simulink model "LCK_0112"  (R2018b)
settings: Solver=FixedStepDiscrete  StartTime=0.0  StopTime=inf  FixedStep=0.01  RelTol=1e-3
PostLoadFcn:
  | if any(exist('dsrtsu_mdlpostloadfcn', 'file') ~= 0), dsrtsu_mdlpostloadfcn('Execute', bdroot); end
values from neighbouring files (symbols this model uses):
  C_DEG2RAD = 0.0175    [LCK_Macro.sldd]
  C_KPH2MPS = 0.2778    [LCK_Macro.sldd]
  C_NEARZERO = 0.0001    [LCK_Macro.sldd]
  C_ONE = 1.0    [LCK_Macro.sldd]
  C_RAD2DEG = 57.2958    [LCK_Macro.sldd]
  C_ZERO = 0.0    [LCK_Macro.sldd]
  k_accel_pedal_pos_per_speed_x : value not decoded    [LCK_LogicPara.sldd]
  k_accel_pedal_pos_per_speed_z : value not decoded    [LCK_LogicPara.sldd]
  k_brake_suprress_hold = 1000.0    [LCK_LogicPara.sldd]
  k_driver_appl_torque_filt = 50.0    [LCK_LogicPara.sldd]
  k_driver_suppression_hold_time = 3000.0    [LCK_LogicPara.sldd]
  k_hands_on_wheel_hold_msec = 500.0    [LCK_LogicPara.sldd]
  k_hands_on_wheel_torque_hi = 0.2    [LCK_LogicPara.sldd]
  k_hands_on_wheel_torque_lo = 0.15    [LCK_LogicPara.sldd]
  k_handsoff_delay_cycles = 50.0    [LCK_LogicPara.sldd]
  k_handsoff_torq_Lo_CR = 0.3    [LCK_LogicPara.sldd]
  k_handson_delay_cycles = 5.0    [LCK_LogicPara.sldd]
  k_HighAccel_suppress_hold = 3000.0    [LCK_LogicPara.sldd]
  k_HLR_suprress_hold = 3000.0    [LCK_LogicPara.sldd]
  k_hs_StrAng_CR_threshold_z : value not decoded    [LCK_LogicPara.sldd]
  k_LC_Exit_Switch = 0.0    [LCK_LogicPara.sldd]
  k_LCG_Configured = 1.0    [LCK_LogicPara.sldd]
  k_LCK_A0_Rdy2Act_UseConst = 0.0    [LCK_LogicPara.sldd]
  k_LCK_A0Fac_ActSta : value not decoded    [LCK_CtrlPara.sldd]
  k_LCK_A0Fac_DrvStm : value not decoded    [LCK_CtrlPara.sldd]
  k_LCK_A0Shift_LftCurv : value not decoded    [LCK_CtrlPara.sldd]
  k_LCK_A0Shift_RgtCurv : value not decoded    [LCK_CtrlPara.sldd]
  k_LCK_A0Shift_StraLan = 0.0    [LCK_CtrlPara.sldd]
  k_LCK_A0ShiftFac_Dy_LftCurv : value not decoded    [LCK_CtrlPara.sldd]
  k_LCK_A0ShiftFac_Dy_RgtCurv : value not decoded    [LCK_CtrlPara.sldd]
  k_LCK_A0ShiftFac_Vspd : value not decoded    [LCK_CtrlPara.sldd]
  k_LCK_accel_inhibit_thold = 35.0    [LCK_LogicPara.sldd]
  k_LCK_Active2Ready_Mask = 255.0    [LCK_LogicPara.sldd]
  k_LCK_CvatRateBks : value not decoded    [LCK_CtrlPara.sldd]
  k_LCK_CvatrBks : value not decoded    [LCK_CtrlPara.sldd]
  k_LCK_DFac_Dy : value not decoded    [LCK_CtrlPara.sldd]
  k_LCK_DFac_Dy_Curv : value not decoded    [LCK_CtrlPara.sldd]
  k_LCK_DFac_HaCurCen : value not decoded    [LCK_CtrlPara.sldd]
  k_LCK_DFac_HaCurSid : value not decoded    [LCK_CtrlPara.sldd]
  k_LCK_DFac_HadCurCen : value not decoded    [LCK_CtrlPara.sldd]
  k_LCK_DFac_HadCurSid : value not decoded    [LCK_CtrlPara.sldd]
  k_LCK_DFac_HadStrCen : value not decoded    [LCK_CtrlPara.sldd]
  k_LCK_DFac_HadStrSid : value not decoded    [LCK_CtrlPara.sldd]
  k_LCK_DFac_HaStrCen : value not decoded    [LCK_CtrlPara.sldd]
  k_LCK_DFac_HaStrSid : value not decoded    [LCK_CtrlPara.sldd]
  k_LCK_DFac_Rad : value not decoded    [LCK_CtrlPara.sldd]
  k_LCK_DFac_SA_CurCen : value not decoded    [LCK_CtrlPara.sldd]
  k_LCK_DFac_SA_CurSid : value not decoded    [LCK_CtrlPara.sldd]
  k_LCK_DFac_SA_StrCen : value not decoded    [LCK_CtrlPara.sldd]
  k_LCK_DFac_SA_StrSid : value not decoded    [LCK_CtrlPara.sldd]
  k_LCK_DFac_SS_CurCen : value not decoded    [LCK_CtrlPara.sldd]
  k_LCK_DFac_SS_CurSid : value not decoded    [LCK_CtrlPara.sldd]
  k_LCK_DFac_SS_StrCen : value not decoded    [LCK_CtrlPara.sldd]
  k_LCK_DFac_SS_StrSid : value not decoded    [LCK_CtrlPara.sldd]
  k_LCK_DFac_Vspd : value not decoded    [LCK_CtrlPara.sldd]
  k_LCK_DlyTm_DrvStim = 0.2    [LCK_CtrlPara.sldd]
  k_LCK_DTermMax = 2.0    [LCK_CtrlPara.sldd]
  k_LCK_DyBks_Curv : value not decoded    [LCK_CtrlPara.sldd]
  k_LCK_Enable_POOnly = 1.0    [LCK_LogicPara.sldd]
  k_LCK_Entry_DistBuffer = 0.1    [LCK_LogicPara.sldd]
  k_LCK_Fac_Vspd2RngThr_FalRec = 0.23    [LCK_CtrlPara.sldd]
  k_LCK_Ffw_CvatSwh = 0.0    [LCK_CtrlPara.sldd]
  k_LCK_Ffw_DyBks : value not decoded    [LCK_CtrlPara.sldd]
  k_LCK_Ffw_TimCon_CmdFlt = 0.0    [LCK_CtrlPara.sldd]
  k_LCK_FfwDeltaFac_Rad_Lft : value not decoded    [LCK_CtrlPara.sldd]
  k_LCK_FfwDeltaFac_Rad_Rgt : value not decoded    [LCK_CtrlPara.sldd]
  k_LCK_FfwDeltaFac_Vspd : value not decoded    [LCK_CtrlPara.sldd]
  k_LCK_FfwFac_CvatRate_Lft : value not decoded    [LCK_CtrlPara.sldd]
  k_LCK_FfwFac_CvatRate_Rgt : value not decoded    [LCK_CtrlPara.sldd]
  k_LCK_FfwFac_Dy : value not decoded    [LCK_CtrlPara.sldd]
  k_LCK_FfwFac_Rad_Lft : value not decoded    [LCK_CtrlPara.sldd]
  k_LCK_FfwFac_Rad_Rgt : value not decoded    [LCK_CtrlPara.sldd]
  k_LCK_FfwFac_Vspd : value not decoded    [LCK_CtrlPara.sldd]
  k_LCK_FfwTorq_Cvat : value not decoded    [LCK_CtrlPara.sldd]
  k_LCK_HAFac_ActSta : value not decoded    [LCK_CtrlPara.sldd]
  k_LCK_HAFac_DrvStm : value not decoded    [LCK_CtrlPara.sldd]
  k_LCK_HaloTime = 2000.0    [LCK_LogicPara.sldd]
  k_LCK_HaloTime_Switch = 0.0    [LCK_LogicPara.sldd]
  k_LCK_HARFac_ActSta : value not decoded    [LCK_CtrlPara.sldd]
  k_LCK_HARFac_DrvStm : value not decoded    [LCK_CtrlPara.sldd]
  k_LCK_Hed_DyBks : value not decoded    [LCK_CtrlPara.sldd]
  k_LCK_HedAngDiffX : value not decoded    [LCK_CtrlPara.sldd]
  k_LCK_HedAngRateDiffX : value not decoded    [LCK_CtrlPara.sldd]
  k_LCK_HndsOnWhel_DlyTm_Idl2Rdy = 0.0    [LCK_LogicPara.sldd]
  k_LCK_host_veh_width = 1.86    [LCK_LogicPara.sldd]
  k_LCK_Idle2Ready_Mask = 239.0    [LCK_LogicPara.sldd]
  k_LCK_Junc_SusTime = 1.0    [LCK_LogicPara.sldd]
  k_LCK_KpKdDecSlopeLmt = 10.0    [LCK_CtrlPara.sldd]
  k_LCK_KpKdIncSlopeLmt = 5.0    [LCK_CtrlPara.sldd]
  k_LCK_Lat_Ctrl_DFac_Lft = 1.0    [LCK_CtrlPara.sldd]
  k_LCK_Lat_Ctrl_DFac_Rgt = 1.05    [LCK_CtrlPara.sldd]
  k_LCK_Lat_Ctrl_Kd = 0.8    [LCK_CtrlPara.sldd]
  k_LCK_Lat_Ctrl_Ki = 0.5    [LCK_CtrlPara.sldd]
  k_LCK_Lat_Ctrl_Kp = 0.7    [LCK_CtrlPara.sldd]
  k_LCK_Lat_Ctrl_Kp_NearGain = 0.7    [LCK_CtrlPara.sldd]
  k_LCK_Lat_Ctrl_PFac_Lft = 1.0    [LCK_CtrlPara.sldd]
  k_LCK_Lat_Ctrl_PFac_Rgt = 1.05    [LCK_CtrlPara.sldd]
  k_LCK_Lat_Ctrl_TimCon_CmdFlt = 5.0    [LCK_CtrlPara.sldd]
  k_LCK_Lat_DFac_Rad : value not decoded    [LCK_CtrlPara.sldd]
  k_LCK_Lat_DFac_SS_Cur : value not decoded    [LCK_CtrlPara.sldd]
  k_LCK_Lat_DFac_SS_Str : value not decoded    [LCK_CtrlPara.sldd]
  k_LCK_Lat_DFac_Vspd : value not decoded    [LCK_CtrlPara.sldd]
  k_LCK_Lat_DyBks : value not decoded    [LCK_CtrlPara.sldd]
  k_LCK_Lat_IFac_Rad : value not decoded    [LCK_CtrlPara.sldd]
  k_LCK_Lat_IFac_Vspd : value not decoded    [LCK_CtrlPara.sldd]
  k_LCK_Lat_ILmtFac_Dy_CurvLan : value not decoded    [LCK_CtrlPara.sldd]
  k_LCK_Lat_ILmtFac_Dy_StraLan : value not decoded    [LCK_CtrlPara.sldd]
  k_LCK_Lat_ILmtFac_Rad : value not decoded    [LCK_CtrlPara.sldd]
  k_LCK_Lat_ILmtFac_Rad_NearGain = 1.0    [LCK_CtrlPara.sldd]
  k_LCK_Lat_ILmtFac_Vspd_CurvLan : value not decoded    [LCK_CtrlPara.sldd]
  k_LCK_Lat_ILmtFac_Vspd_StraLan : value not decoded    [LCK_CtrlPara.sldd]
  k_LCK_Lat_ITermLmt_Dy = 1.0    [LCK_CtrlPara.sldd]
  k_LCK_Lat_KpKdDecSlopeLmt = 10.0    [LCK_CtrlPara.sldd]
  k_LCK_Lat_KpKdIncSlopeLmt = 10.0    [LCK_CtrlPara.sldd]
  k_LCK_Lat_PFac_Dy_InnLftCur : value not decoded    [LCK_CtrlPara.sldd]
  k_LCK_Lat_PFac_Dy_InnRgtCur : value not decoded    [LCK_CtrlPara.sldd]
  k_LCK_Lat_PFac_Dy_OutLftCur : value not decoded    [LCK_CtrlPara.sldd]
  k_LCK_Lat_PFac_Dy_OutRgtCur : value not decoded    [LCK_CtrlPara.sldd]
  k_LCK_Lat_PFac_Dy_Str : value not decoded    [LCK_CtrlPara.sldd]
  k_LCK_Lat_PFac_Rad : value not decoded    [LCK_CtrlPara.sldd]
  ... (+153 more)
undefined symbols (not defined in the file or in its folder): k_LCK_CurvBks, K_LCK_SPA0A1A2_LMRngCmp_y
libraries: LateralControl_fcns_lib x58, simulink x24
(part 21 of 45)

== system LCK_0112/Lateral_Control_Module/Adas_Lateral_Control_LCK_Core/Module 9/Module 0 ==
  Hed_Ang : Inport
  Hed_Ang_Diff_Rat : Inport  Port=2
  Dy_0 : Inport  Port=3
  Str_Flag : Inport  Port=4
  Vspd : Inport  Port=5
  Road_Radius : Inport  Port=6
  Steer_Ang : Inport  Port=7
  Steer_Spd : Inport  Port=8
  Cen_Flag : Inport  Port=9
  Bus Creator{1..8} (8 alike) : BusCreator  Inputs=2
  Bus Selector{1..7,11} (8 alike) : BusSelector  OutputSignals=signal1
  Bus Selector{8..10,12..16} (8 alike) : BusSelector  OutputSignals=signal2
  D Gain : Subsystem
  "Definition Fac 1 " : Subsystem
  Definition Fac 2 : Subsystem
  Definition Fac 3 : Subsystem
  Definition Fac 4 : Subsystem
  Definition Fac 5 : Subsystem
  Definition Fac 6 : Subsystem
  Definition Fac 7 : Subsystem
  Definition Fac 8 : Subsystem
  Limitation of D Gain : Subsystem
  Limitation of P Gain : Subsystem
  P Gain : Subsystem
  P_Gain : Outport
  D_Gain : Outport  Port=2
  wires:
  Limitation of P Gain/1(P_Gain_Limited) -> P_Gain/1
  Limitation of D Gain/1(D_Gain_Limited) -> D_Gain/1
  Hed_Ang/1 -> "Definition Fac 1 "/1(Hed_Ang), Definition Fac 2/1(Hed_Ang)
  Hed_Ang_Diff_Rat/1 -> "Definition Fac 1 "/2(Hed_Ang_Diff_Rat), Definition Fac 3/1(Hed_Ang_Diff_Rat)
  Cen_Flag/1 -> Definition Fac 3/2(Cen_Flag), Definition Fac 5/2(Cen_Flag), Definition Fac 4/2(Cen_Flag), Definition Fac 2/2(Cen_Flag)
  Str_Flag/1 -> Definition Fac 3/3(Str_Flag), Definition Fac 6/1(Str_Flag), Definition Fac 5/3(Str_Flag), Definition Fac 4/3(Str_Flag), Definition Fac 2/3(Str_Flag)
  Steer_Ang/1 -> Definition Fac 4/1(Steer_Ang)
  Steer_Spd/1 -> Definition Fac 5/1(Steer_Spd)
  Dy_0/1 -> Definition Fac 6/2(Dy_0)
  Vspd/1 -> Definition Fac 7/1(Vspd)
  Road_Radius/1 -> Definition Fac 8/1(Road_Radius)
  P Gain/1(P_Gain) -> Limitation of P Gain/1(P_Gain)
  "Definition Fac 1 "/1(LatCtrl_PFac_Asym) -> Bus Creator4/1
  "Definition Fac 1 "/2(LatCtrl_DFac_Asym) -> Bus Creator4/2
  Definition Fac 2/1(LatCtrl_PFac_HedAngDiff) -> Bus Creator1/1
  Definition Fac 2/2(LatCtrl_DFac_HedAngDiff) -> Bus Creator1/2
  Definition Fac 3/1(LatCtrl_PFac_HedAngDiffRat) -> Bus Creator2/1
  Definition Fac 3/2(LatCtrl_DFac_HedAngDiffRat) -> Bus Creator2/2
  Definition Fac 4/1(LatCtrl_PFac_StrAng) -> Bus Creator3/1
  Definition Fac 4/2(LatCtrl_DFac_StrAng) -> Bus Creator3/2
  Definition Fac 5/1(LatCtrl_PFac_StrSpd) -> Bus Creator5/1
  Definition Fac 5/2(LatCtrl_DFac_StrSpd) -> Bus Creator5/2
  Definition Fac 6/1(LatCtrl_PFac_Dy) -> Bus Creator6/1
  Definition Fac 6/2(LatCtrl_DFac_Dy) -> Bus Creator6/2
  Definition Fac 7/1(LatCtrl_PFac_Vspd) -> Bus Creator7/1
  Definition Fac 7/2(LatCtrl_DFac_Vspd) -> Bus Creator7/2
  Definition Fac 8/1(HedCtrl_PFac_Radius) -> Bus Creator8/1
  Definition Fac 8/2(HedCtrl_DFac_Radius) -> Bus Creator8/2
  Bus Selector11/1 -> P Gain/1(LatCtrl_PFac_Asym)  "<signal1>"
  Bus Creator4/1 -> Bus Selector8/1, Bus Selector11/1
  Bus Selector1/1 -> P Gain/2(LatCtrl_PFac_HedAngDiff)  "<signal1>"
  Bus Creator1/1 -> Bus Selector9/1, Bus Selector1/1
  Bus Selector2/1 -> P Gain/3(LatCtrl_PFac_HedAngDiffRat)  "<signal1>"
  Bus Creator2/1 -> Bus Selector10/1, Bus Selector2/1
  Bus Selector3/1 -> P Gain/4(LatCtrl_PFac_StrAng)  "<signal1>"
  Bus Creator3/1 -> Bus Selector3/1, Bus Selector12/1
  Bus Selector4/1 -> P Gain/5(LatCtrl_PFac_StrSpd)  "<signal1>"
  Bus Creator5/1 -> Bus Selector4/1, Bus Selector13/1
  Bus Selector5/1 -> P Gain/6(LatCtrl_PFac_Dy)  "<signal1>"
  Bus Creator6/1 -> Bus Selector5/1, Bus Selector14/1
  Bus Selector6/1 -> P Gain/7(LatCtrl_PFac_Vspd)  "<signal1>"
  Bus Creator7/1 -> Bus Selector6/1, Bus Selector15/1
  Bus Selector7/1 -> P Gain/8(LatCtrl_PFac_Radius)  "<signal1>"
  Bus Creator8/1 -> Bus Selector16/1, Bus Selector7/1
  D Gain/1(D_Gain) -> Limitation of D Gain/1(D_Gain)
  Bus Selector8/1 -> D Gain/1(LatCtrl_DFac_Asym)  "<signal2>"
  Bus Selector9/1 -> D Gain/2(LatCtrl_DFac_HedAngDiff)  "<signal2>"
  Bus Selector10/1 -> D Gain/3(LatCtrl_DFac_HedAngDiffRat)  "<signal2>"
  Bus Selector12/1 -> D Gain/4(LatCtrl_DFac_StrAng)  "<signal2>"
  Bus Selector13/1 -> D Gain/5(LatCtrl_DFac_StrSpd)  "<signal2>"
  Bus Selector14/1 -> D Gain/6(LatCtrl_DFac_Dy)  "<signal2>"
  Bus Selector15/1 -> D Gain/7(LatCtrl_DFac_Vspd)  "<signal2>"
  Bus Selector16/1 -> D Gain/8(LatCtrl_DFac_Radius)  "<signal2>"

== system LCK_0112/Lateral_Control_Module/Adas_Lateral_Control_LCK_Core/Module 9/Module 1 ==
  Hed_Ang : Inport
  Hed_Ang_Rat : Inport  Port=2
  P_Gain : Inport  Port=3
  D_Gain : Inport  Port=4
  Add : Sum
  First_Order_Lag_Filter_LIB : LateralControl_fcns_lib/First_Order_Lag_Filter_LIB  SystemSampleTime=-1
  Gain{,1,3..4} (4 alike) : Gain  Gain=-1
  ML_TIME_MSEC2 : Constant  Description=_GWMAB30P3.LCK.000_166_  Value=ML_TIME_MSEC
  Product : Product
  Product2 : Product
  Saturation : Saturate  UpperLimit=3  LowerLimit=-3  OutDataTypeStr=Inherit: Inherit via back propagation
  Saturation Dynamic : simulink/Discontinuities/Saturation Dynamic  OutMin=[]  OutMax=[]  OutDataTypeStr=Inherit: Same as second input  OutDataType=fixdt(1, 16)  OutScaling=2^-10  DoSatur=off
  Saturation Dynamic1 : simulink/Discontinuities/Saturation Dynamic  OutMin=[]  OutMax=[]  OutDataTypeStr=Inherit: Same as second input  OutDataType=fixdt(1, 16)  OutScaling=2^-10  DoSatur=off
  k_LCK_DTermMax : Constant  Value=k_LCK_DTermMax
  k_LCK_LatCtrl_TimCon_CmdFlt : Constant  Description=_GWMAB30P3.LCK.000_168_  Value=k_LCK_LatCtrl_TimCon_CmdFlt
  k_LCK_PTermMax : Constant  Value=k_LCK_PTermMax
  LatCtrl_Cmd : Outport
  LatCtrl_P_Term : Outport  Port=2
  LatCtrl_D_Term : Outport  Port=3
  wires:
  Gain4/1 -> Saturation Dynamic1/3
  k_LCK_DTermMax/1 -> Saturation Dynamic1/1, Gain4/1
  Saturation Dynamic1/1 -> Add/2, LatCtrl_D_Term/1
  Product2/1 -> Saturation Dynamic1/2
  D_Gain/1 -> Gain3/1
  Hed_Ang_Rat/1 -> Product2/1
  Saturation/1 -> LatCtrl_Cmd/1
  P_Gain/1 -> Gain1/1
  Hed_Ang/1 -> Product/2
  Product/1 -> Saturation Dynamic/2
  Saturation Dynamic/1 -> Add/1, LatCtrl_P_Term/1
  k_LCK_PTermMax/1 -> Gain/1, Saturation Dynamic/1
  Gain/1 -> Saturation Dynamic/3
  Add/1 -> First_Order_Lag_Filter_LIB/1
  First_Order_Lag_Filter_LIB/1 -> Saturation/1
  k_LCK_LatCtrl_TimCon_CmdFlt/1 -> First_Order_Lag_Filter_LIB/2
  ML_TIME_MSEC2/1 -> First_Order_Lag_Filter_LIB/3
  Gain1/1 -> Product/1
  Gain3/1 -> Product2/2
